simulink model "UNIVERSAL_MOTOR"  (R2021a)
settings: Solver=VariableStepAuto  StartTime=0.0  StopTime=1  RelTol=1e-3
settings Model: Creator=SA  LastModifiedBy=SA

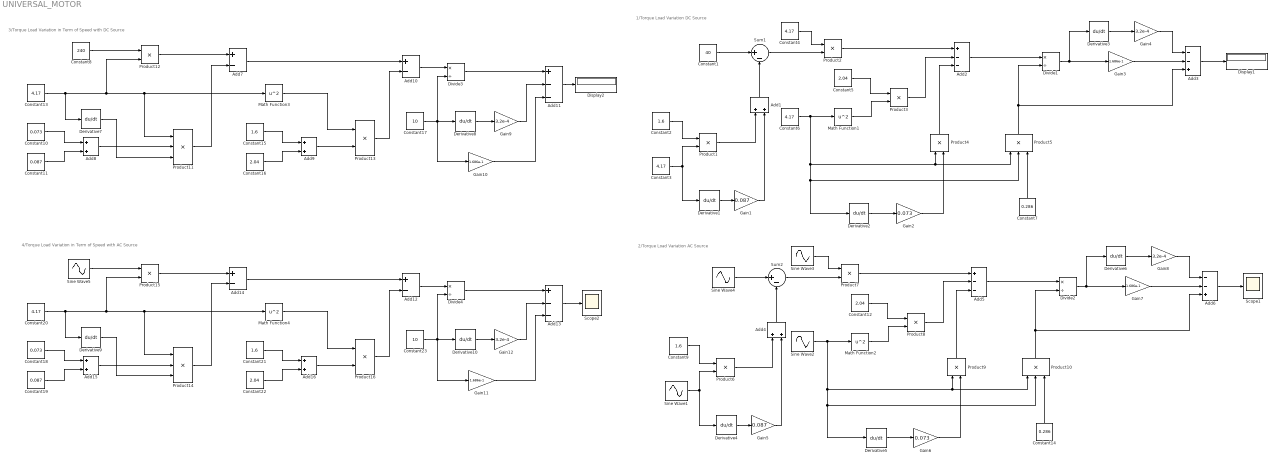
== system UNIVERSAL_MOTOR ==
  note: 4/Torque Load Variation in Term of Speed with AC Source
  note: 3/Torque Load Variation in Term of Speed with DC Source
  note: 2/Torque Load Variation AC Source
  note: 1/Torque Load Variation DC Source
  Add{1,4,8..9,15..16} (6 alike) : Sum
  Add{7,10,12,14} (4 alike) : Sum  Inputs=+-
  Add{2,5,11,13} (4 alike) : Sum  Inputs=+--
  Add3 : Sum  Inputs=--+
  Add6 : Sum  Inputs=--+
  Constant1 : Constant  Value=40
  Constant10 : Constant  Value=0.073
  Constant11 : Constant  Value=0.087
  Constant{5,12,16,22} (4 alike) : Constant  Value=2.04
  Constant{3..4,6,13,20} (5 alike) : Constant  Value=4.17
  Constant14 : Constant  Value=0.286
  Constant{2,9,15,21} (4 alike) : Constant  Value=1.6
  Constant17 : Constant  Value=10
  Constant18 : Constant  Value=0.073
  Constant19 : Constant  Value=0.087
  Constant23 : Constant  Value=10
  Constant7 : Constant  Value=0.286
  Constant8 : Constant  Value=240
  Derivative{1..10} (10 alike) : Derivative
  Display1 : Display
  Display2 : Display
  Divide{1..4} (4 alike) : Product  Inputs=*/
  Gain1 : Gain  Gain=0.087
  Gain{3,7,10..11} (4 alike) : Gain  Gain=1.686e-1
  Gain{4,8..9,12} (4 alike) : Gain  Gain=3.2e-4
  Gain2 : Gain  Gain=0.073
  Gain5 : Gain  Gain=0.087
  Gain6 : Gain  Gain=0.073
  Math Function{1..4} (4 alike) : Math  Operator=square  SaturateOnIntegerOverflow=on
  Product{1..4,6..9,12..13,15..16} (12 alike) : Product
  Product{5,10..11,14} (4 alike) : Product  Inputs=3
  Scope1 : Scope
  Scope2 : Scope
  Sine Wave1 : Sin  Amplitude=4.17  Frequency=60  SampleTime=0
  Sine Wave2 : Sin  Amplitude=4.17  Frequency=60  SampleTime=0
  Sine Wave3 : Sin  Amplitude=4.17  Frequency=60  SampleTime=0
  Sine Wave4 : Sin  Amplitude=20  Frequency=60  SampleTime=0
  Sine Wave5 : Sin  Amplitude=20  Frequency=60  SampleTime=0
  Sum1 : Sum  Inputs=|+-
  Sum2 : Sum  Inputs=|+-
  wires:
  Add1/1 -> Sum1/2
  Constant1/1 -> Sum1/1
  Product1/1 -> Add1/1
  Constant2/1 -> Product1/1
  Constant3/1 -> Product1/2, Derivative1/1
  Derivative1/1 -> Gain1/1
  Gain1/1 -> Add1/2
  Sum1/1 -> Product2/2
  Constant4/1 -> Product2/1
  Product2/1 -> Add2/1
  Product3/1 -> Add2/2
  Constant5/1 -> Product3/1
  Math Function1/1 -> Product3/2
  Constant6/1 -> Product5/2, Derivative2/1, Product5/1, Product4/1, Math Function1/1
  Product4/1 -> Add2/3
  Derivative2/1 -> Gain2/1
  Gain2/1 -> Product4/2
  Add2/1 -> Divide1/1
  Constant7/1 -> Product5/3
  Gain3/1 -> Add3/2
  Divide1/1 -> Derivative3/1, Gain3/1
  Derivative3/1 -> Gain4/1
  Gain4/1 -> Add3/1
  Product5/1 -> Add3/3, Divide1/2
  Add3/1 -> Display1/1
  Add4/1 -> Sum2/2
  Product10/1 -> Add6/3, Divide2/2
  Gain5/1 -> Add4/2
  Sum2/1 -> Product7/2
  Sine Wave3/1 -> Product7/1
  Derivative4/1 -> Gain5/1
  Add5/1 -> Divide2/1
  Derivative5/1 -> Gain6/1
  Sine Wave2/1 -> Product10/2, Derivative5/1, Product10/1, Product9/1, Math Function2/1
  Sine Wave4/1 -> Sum2/1
  Gain7/1 -> Add6/2
  Math Function2/1 -> Product8/2
  Product8/1 -> Add5/2
  Add6/1 -> Scope1/1
  Constant14/1 -> Product10/3
  Product6/1 -> Add4/1
  Gain6/1 -> Product9/2
  Product9/1 -> Add5/3
  Constant9/1 -> Product6/1
  Constant12/1 -> Product8/1
  Gain8/1 -> Add6/1
  Product7/1 -> Add5/1
  Sine Wave1/1 -> Product6/2, Derivative4/1
  Divide2/1 -> Derivative6/1, Gain7/1
  Derivative6/1 -> Gain8/1
  Constant8/1 -> Product12/1
  Product12/1 -> Add7/1
  Add8/1 -> Product11/2
  Product11/1 -> Add7/2
  Constant10/1 -> Add8/1
  Constant11/1 -> Add8/2
  Constant13/1 -> Derivative7/1, Product11/1, Math Function3/1, Product12/2
  Derivative7/1 -> Product11/3
  Constant16/1 -> Add9/2
  Constant15/1 -> Add9/1
  Add9/1 -> Product13/2
  Math Function3/1 -> Product13/1
  Add7/1 -> Add10/1
  Product13/1 -> Add10/2
  Add10/1 -> Divide3/1
  Divide3/1 -> Add11/1
  Constant17/1 -> Gain10/1, Divide3/2, Derivative8/1
  Derivative8/1 -> Gain9/1
  Gain9/1 -> Add11/2
  Gain10/1 -> Add11/3
  Add11/1 -> Display2/1
  Derivative10/1 -> Gain12/1
  Add13/1 -> Scope2/1
  Add15/1 -> Product14/2
  Constant19/1 -> Add15/2
  Divide4/1 -> Add13/1
  Constant18/1 -> Add15/1
  Constant21/1 -> Add16/1
  Constant22/1 -> Add16/2
  Add16/1 -> Product16/2
  Sine Wave5/1 -> Product15/1
  Math Function4/1 -> Product16/1
  Constant23/1 -> Gain11/1, Divide4/2, Derivative10/1
  Derivative9/1 -> Product14/3
  Product16/1 -> Add12/2
  Constant20/1 -> Derivative9/1, Product14/1, Math Function4/1, Product15/2
  Gain12/1 -> Add13/2
  Add14/1 -> Add12/1
  Product15/1 -> Add14/1
  Product14/1 -> Add14/2
  Gain11/1 -> Add13/3
  Add12/1 -> Divide4/1
